simulink model "motor_testing"  (R2019b)
settings: Solver=VariableStepAuto  StartTime=0.0  StopTime=200  MaxStep=0.01  RelTol=1e-3
InitFcn:
  | Motor_torque_constant = 1.22; % NM/A
  | Kb = (84.5/(1000*2*pi/60)); %or  V/Wm (wm in rps) volt/rps
  | Jm =10.2 *10^-3; %kgm^2
  | Bm = ((Motor_torque_constant)*(25)/(210*2*pi/60));
  | Motor_resistance =244*10^-3; %ohm
  | L = 1.4*10^-3;% H(henry)
  | alpha_Conductor =0.0040;
  | Ref_Temp = 25;
  | Alpha_Magnet = -0.0020;
undefined symbols (not defined in the file or in its folder): sigbuilder_block
settings Model: SimulationMode=accelerator  Creator=Avmash  LastModifiedBy=Avmash

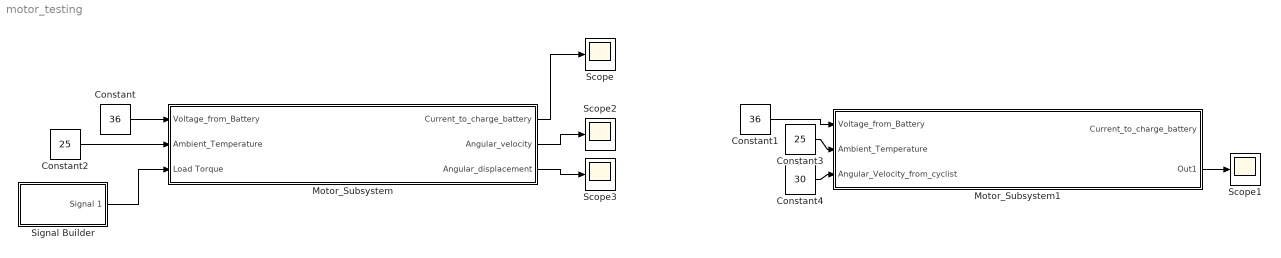
== system motor_testing ==
  Constant : Constant  Value=36
  Constant1 : Constant  Value=36
  Constant2 : Constant  Value=25
  Constant3 : Constant  Value=25
  Constant4 : Constant  Value=30
  Motor_Subsystem : Subsystem
  Motor_Subsystem1 : Subsystem
  Scope{,1..3} (4 alike) : Scope
  Signal Builder : Subsystem  Tag=STV Subsys  LoadFcn=sigbuilder_block('load');  StartFcn=sigbuilder_block('start');  StopFcn=sigbuilder_block('stop');  ClipboardFcn=sigbuilder_block('clipboard');  mask(Sigbuilder block){tuvar=[0:10]}
      mask help: Simulink:masks:SigbuilderBlock_MD
      mask init:
      | if ~strcmp(get_param(bdroot(gcbh),'SimulationStatus'),'stopped') tuvar = sigbuilder_block('maskInit'); end
      settings: CopyFcn=sigbuilder_block('copy');  DeleteFcn=sigbuilder_block('delete');  ModelCloseFcn=sigbuilder_block('modelClose');  PreSaveFcn=sigbuilder_block('preSave');  PauseFcn=sigbuilder_block('pause');  ContinueFcn=sigbuilder_block('continue');  NameChangeFcn=sigbuilder_block('namechange');  OpenFcn=sigbuilder_block('open',[437.6 153 550.4 359.25 ]);  CloseFcn=sigbuilder_block('close');
      mask Display: plot(0, 0, 100, 100,[2, 2, 32, 32, 2], [68, 8, 8, 68, 68],[32, 2], [38, 38], [32, 19, 2],[53, 60, 44], [32, 17, 17, 2],[16, 16, 31, 31]);txt = getActiveGroup(gcbh);text(2, 100, txt,'verticalAlignment', 'top');
  wires:
  Constant/1 -> Motor_Subsystem/1(Voltage_from_Battery)
  Constant2/1 -> Motor_Subsystem/2(Ambient_Temperature)
  Signal Builder/1(Signal 1) -> Motor_Subsystem/3(Load Torque)
  Motor_Subsystem/1(Current_to_charge_battery) -> Scope/1
  Motor_Subsystem/2(Angular_velocity) -> Scope2/1
  Motor_Subsystem/3(Angular_displacement) -> Scope3/1
  Constant1/1 -> Motor_Subsystem1/1(Voltage_from_Battery)
  Constant3/1 -> Motor_Subsystem1/2(Ambient_Temperature)
  Constant4/1 -> Motor_Subsystem1/3(Angular_Velocity_from_cyclist)
  Motor_Subsystem1/2(Out1) -> Scope1/1

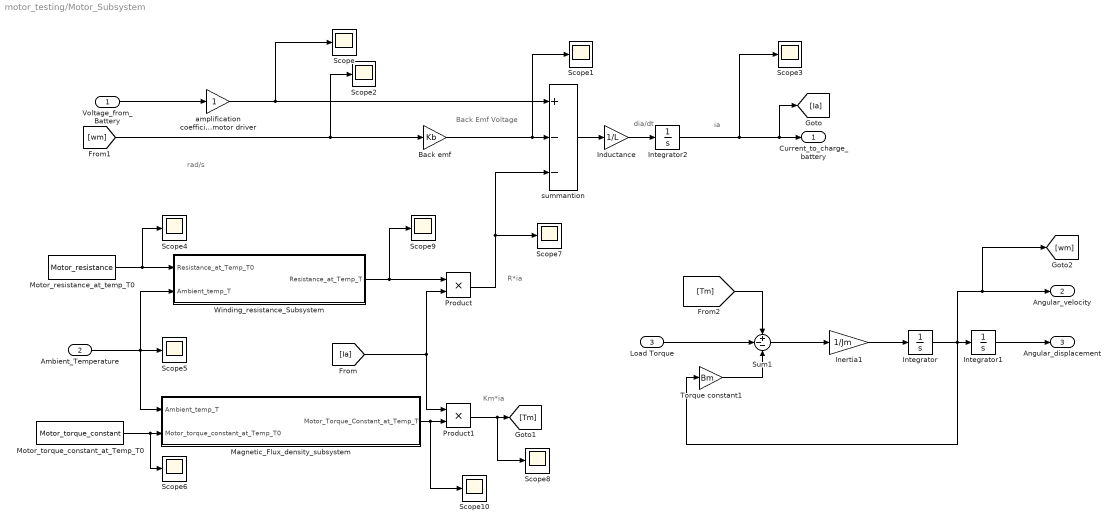
== system motor_testing/Motor_Subsystem ==
  note: ia
  note: dia/dt
  note: rad/s
  note: R*ia
  note: Km*ia
  note: Back Emf Voltage
  Voltage_from_Battery : Inport
  Ambient_Temperature : Inport  Port=2
  Load Torque : Inport  Port=3
  " amplification coefficient of the motor driver" : Gain
  Back emf : Gain  Gain=Kb
  Inductance : Gain  Gain=1/L
  Inertia1 : Gain  Gain=1/Jm
  Integrator : Integrator
  Integrator1 : Integrator
  Integrator2 : Integrator
  Magnetic_Flux_density_subsystem : Subsystem
  Motor_resistance_at_temp_T0 : Constant  Value=Motor_resistance
  Motor_torque_constant_at_Temp_T0 : Constant  Value=Motor_torque_constant
  Product : Product
  Product1 : Product
  Scope{,1..10} (11 alike) : Scope
  Sum1 : Sum  Inputs=+--
  Torque constant1 : Gain  Gain=Bm
  Winding_resistance_Subsystem : Subsystem
  summantion : Sum  Inputs=+--
  Current_to_charge_battery : Outport  VectorParamsAs1DForOutWhenUnconnected=off
  Angular_velocity : Outport  Port=2  VectorParamsAs1DForOutWhenUnconnected=off
  Angular_displacement : Outport  Port=3
  wires:
  Voltage_from_Battery/1 -> " amplification coefficient of the motor driver"/1
  Back emf/1 -> Scope1/1, summantion/2
  Inductance/1 -> Integrator2/1
  summantion/1 -> Inductance/1
  Motor_resistance_at_temp_T0/1 -> Scope4/1, Winding_resistance_Subsystem/1(Resistance_at_Temp_T0)
  Product/1 -> summantion/3, Scope7/1
  Ambient_Temperature/1 -> Winding_resistance_Subsystem/2(Ambient_temp_T), Scope5/1, Magnetic_Flux_density_subsystem/1(Ambient_temp_T)
  Motor_torque_constant_at_Temp_T0/1 -> Scope6/1, Magnetic_Flux_density_subsystem/2(Motor_torque_constant_at_Temp_T0)
  [Ia] -> Product1/1, Product/2
  Magnetic_Flux_density_subsystem/1(Motor_Torque_Constant_at_Temp_T) -> Scope10/1, Product1/2
  Product1/1 -> Scope8/1, [Tm]
  Winding_resistance_Subsystem/1(Resistance_at_Temp_T) -> Scope9/1, Product/1
  [wm] -> Scope2/1, Back emf/1
  Integrator2/1 -> Scope3/1, [Ia], Current_to_charge_battery/1
  " amplification coefficient of the motor driver"/1 -> Scope/1, summantion/1
  [Tm] -> Sum1/1
  Load Torque/1 -> Sum1/2
  Sum1/1 -> Inertia1/1
  Inertia1/1 -> Integrator/1
  Integrator/1 -> [wm], Angular_velocity/1, Torque constant1/1, Integrator1/1
  Integrator1/1 -> Angular_displacement/1
  Torque constant1/1 -> Sum1/3

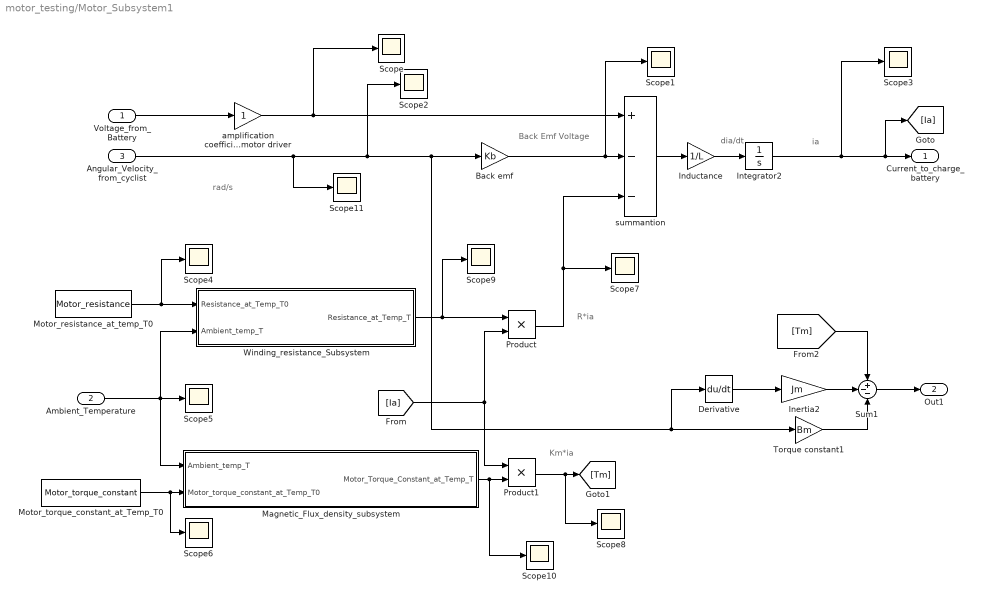
== system motor_testing/Motor_Subsystem1 ==
  note: ia
  note: dia/dt
  note: rad/s
  note: R*ia
  note: Km*ia
  note: Back Emf Voltage
  Voltage_from_Battery : Inport
  Ambient_Temperature : Inport  Port=2
  Angular_Velocity_from_cyclist : Inport  Port=3
  " amplification coefficient of the motor driver" : Gain
  Back emf : Gain  Gain=Kb
  Derivative : Derivative
  Inductance : Gain  Gain=1/L
  Inertia2 : Gain  Gain=Jm
  Integrator2 : Integrator
  Magnetic_Flux_density_subsystem : Subsystem
  Motor_resistance_at_temp_T0 : Constant  Value=Motor_resistance
  Motor_torque_constant_at_Temp_T0 : Constant  Value=Motor_torque_constant
  Product : Product
  Product1 : Product
  Scope{,1..11} (12 alike) : Scope
  Sum1 : Sum  Inputs=+--
  Torque constant1 : Gain  Gain=Bm
  Winding_resistance_Subsystem : Subsystem
  summantion : Sum  Inputs=+--
  Current_to_charge_battery : Outport  VectorParamsAs1DForOutWhenUnconnected=off
  Out1 : Outport  Port=2
  wires:
  Voltage_from_Battery/1 -> " amplification coefficient of the motor driver"/1
  Back emf/1 -> Scope1/1, summantion/2
  Inductance/1 -> Integrator2/1
  summantion/1 -> Inductance/1
  Motor_resistance_at_temp_T0/1 -> Scope4/1, Winding_resistance_Subsystem/1(Resistance_at_Temp_T0)
  Product/1 -> summantion/3, Scope7/1
  Ambient_Temperature/1 -> Winding_resistance_Subsystem/2(Ambient_temp_T), Scope5/1, Magnetic_Flux_density_subsystem/1(Ambient_temp_T)
  Motor_torque_constant_at_Temp_T0/1 -> Scope6/1, Magnetic_Flux_density_subsystem/2(Motor_torque_constant_at_Temp_T0)
  [Ia] -> Product1/1, Product/2
  Magnetic_Flux_density_subsystem/1(Motor_Torque_Constant_at_Temp_T) -> Scope10/1, Product1/2
  Product1/1 -> Scope8/1, [Tm]
  Winding_resistance_Subsystem/1(Resistance_at_Temp_T) -> Scope9/1, Product/1
  Integrator2/1 -> Scope3/1, [Ia], Current_to_charge_battery/1
  " amplification coefficient of the motor driver"/1 -> Scope/1, summantion/1
  [Tm] -> Sum1/1
  Sum1/1 -> Out1/1
  Torque constant1/1 -> Sum1/3
  Inertia2/1 -> Sum1/2
  Derivative/1 -> Inertia2/1
  Angular_Velocity_from_cyclist/1 -> Scope11/1, Scope2/1, Derivative/1, Torque constant1/1, Back emf/1

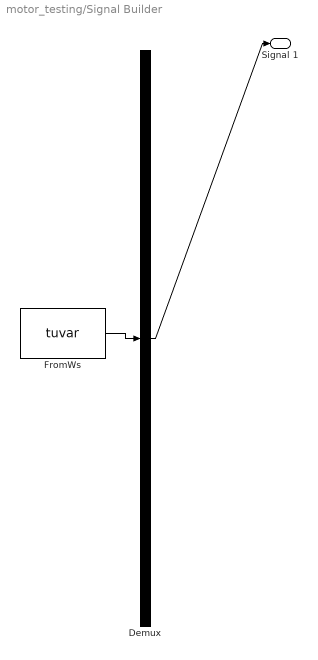
== system motor_testing/Signal Builder ==
  Demux : Demux  Tag=STV Demux  Outputs=1
  FromWs : FromWorkspace  Tag=STV FromWs  VariableName=tuvar  SampleTime=0
      SigBuilderData=|
      | common.afterFinalStr = 'Extrapolate'
      | common.sampleTime = 0
      | dataSet.timeRange = [0 200]
      | dataSet.name = 'Group 1'
      | sbobj.Groups.Name = 'Group 1'
      | sbobj.Groups.Signals.Name = 'Signal 1'
      | sbobj.Groups.Signals.XData = [0 100 100 200]
      | sbobj.Groups.Signals.YData = [0 0 30 30]
      | sbobj.Groups.TimeRange = [0 200]
  Signal 1 : Outport  Tag=STV Outport
  wires:
  FromWs/1 -> Demux/1
  Demux/1 -> Signal 1/1

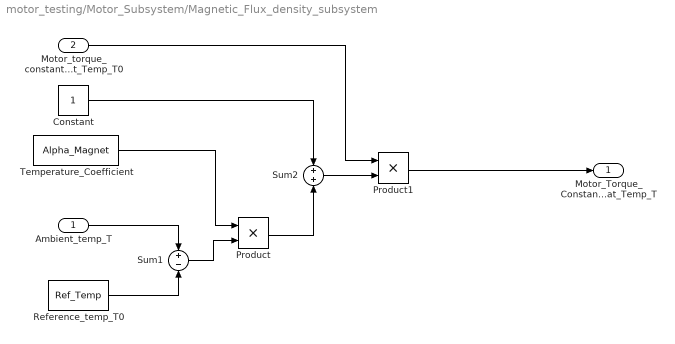
== system motor_testing/Motor_Subsystem/Magnetic_Flux_density_subsystem ==
  Ambient_temp_T : Inport
  Motor_torque_constant_at_Temp_T0 : Inport  Port=2
  Constant : Constant
  Product : Product
  Product1 : Product
  Reference_temp_T0 : Constant  Value=Ref_Temp
  Sum1 : Sum  Inputs=+-
  Sum2 : Sum
  Temperature_Coefficient : Constant  Value=Alpha_Magnet
  Motor_Torque_Constant_at_Temp_T : Outport  VectorParamsAs1DForOutWhenUnconnected=off
  wires:
  Motor_torque_constant_at_Temp_T0/1 -> Product1/1
  Product1/1 -> Motor_Torque_Constant_at_Temp_T/1
  Product/1 -> Sum2/2
  Constant/1 -> Sum2/1
  Sum2/1 -> Product1/2
  Temperature_Coefficient/1 -> Product/1
  Ambient_temp_T/1 -> Sum1/1
  Reference_temp_T0/1 -> Sum1/2
  Sum1/1 -> Product/2

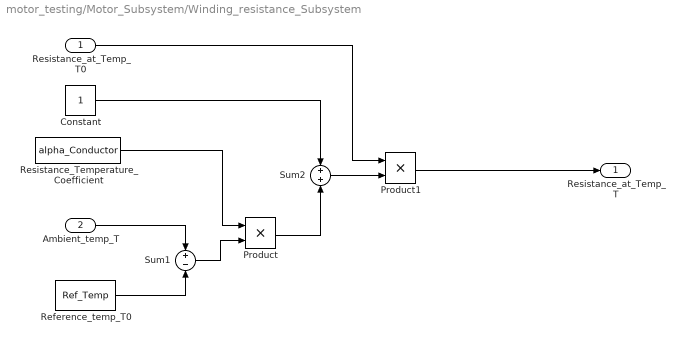
== system motor_testing/Motor_Subsystem/Winding_resistance_Subsystem ==
  Resistance_at_Temp_T0 : Inport
  Ambient_temp_T : Inport  Port=2
  Constant : Constant
  Product : Product
  Product1 : Product
  Reference_temp_T0 : Constant  Value=Ref_Temp
  Resistance_Temperature_Coefficient : Constant  Value=alpha_Conductor
  Sum1 : Sum  Inputs=+-
  Sum2 : Sum
  Resistance_at_Temp_T : Outport  VectorParamsAs1DForOutWhenUnconnected=off
  wires:
  Sum1/1 -> Product/2
  Reference_temp_T0/1 -> Sum1/2
  Ambient_temp_T/1 -> Sum1/1
  Resistance_Temperature_Coefficient/1 -> Product/1
  Sum2/1 -> Product1/2
  Constant/1 -> Sum2/1
  Product/1 -> Sum2/2
  Product1/1 -> Resistance_at_Temp_T/1
  Resistance_at_Temp_T0/1 -> Product1/1

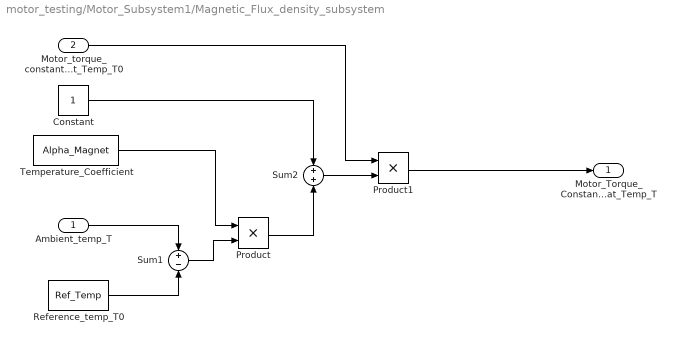
== system motor_testing/Motor_Subsystem1/Magnetic_Flux_density_subsystem ==
  Ambient_temp_T : Inport
  Motor_torque_constant_at_Temp_T0 : Inport  Port=2
  Constant : Constant
  Product : Product
  Product1 : Product
  Reference_temp_T0 : Constant  Value=Ref_Temp
  Sum1 : Sum  Inputs=+-
  Sum2 : Sum
  Temperature_Coefficient : Constant  Value=Alpha_Magnet
  Motor_Torque_Constant_at_Temp_T : Outport  VectorParamsAs1DForOutWhenUnconnected=off
  wires:
  Motor_torque_constant_at_Temp_T0/1 -> Product1/1
  Product1/1 -> Motor_Torque_Constant_at_Temp_T/1
  Product/1 -> Sum2/2
  Constant/1 -> Sum2/1
  Sum2/1 -> Product1/2
  Temperature_Coefficient/1 -> Product/1
  Ambient_temp_T/1 -> Sum1/1
  Reference_temp_T0/1 -> Sum1/2
  Sum1/1 -> Product/2

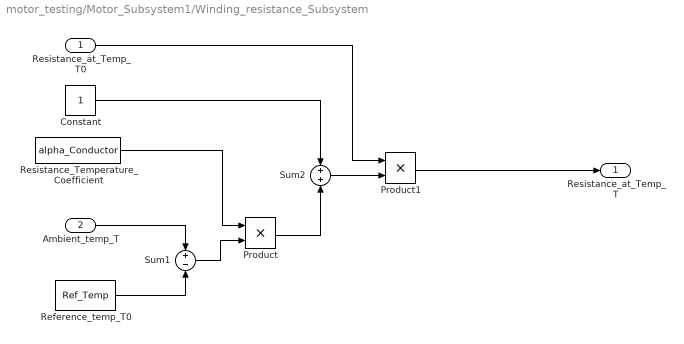
== system motor_testing/Motor_Subsystem1/Winding_resistance_Subsystem ==
  Resistance_at_Temp_T0 : Inport
  Ambient_temp_T : Inport  Port=2
  Constant : Constant
  Product : Product
  Product1 : Product
  Reference_temp_T0 : Constant  Value=Ref_Temp
  Resistance_Temperature_Coefficient : Constant  Value=alpha_Conductor
  Sum1 : Sum  Inputs=+-
  Sum2 : Sum
  Resistance_at_Temp_T : Outport  VectorParamsAs1DForOutWhenUnconnected=off
  wires:
  Sum1/1 -> Product/2
  Reference_temp_T0/1 -> Sum1/2
  Ambient_temp_T/1 -> Sum1/1
  Resistance_Temperature_Coefficient/1 -> Product/1
  Sum2/1 -> Product1/2
  Constant/1 -> Sum2/1
  Product/1 -> Sum2/2
  Product1/1 -> Resistance_at_Temp_T/1
  Resistance_at_Temp_T0/1 -> Product1/1
